simulink model "Task_2"  (R2021b)
settings: Solver=ode23tb  StartTime=0.0  StopTime=1000*3600  RelTol=1e-3
undefined symbols (not defined in the file): Ion, Lithium
libraries: eeStairGenerator x2, spsBatteryLib x1, spsControlledCurrentSourceLib x1, spspowerguiLib x1
settings Model: Creator=eee  LastModifiedBy=casum

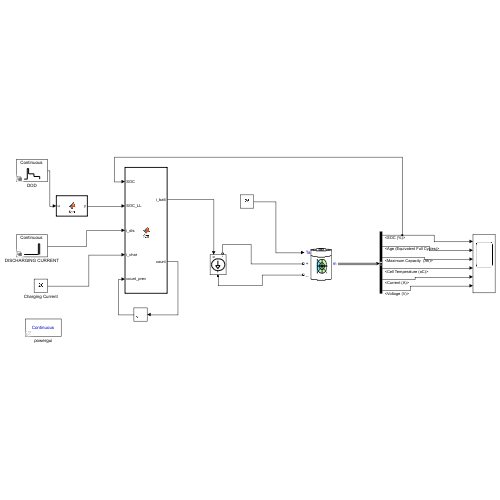
[thumbnail: Simulink's stored preview of the top-level diagram]
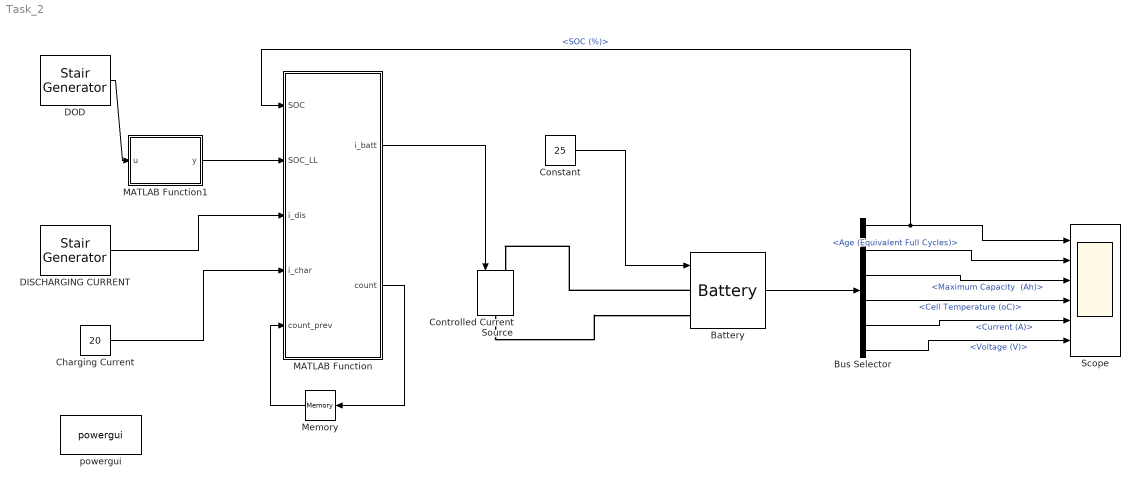
== system Task_2 ==
  Battery : spsBatteryLib/Battery  BatType=Lithium-Ion  ShowTempParam=on  ThermalPreset="12.8V  40Ah  (LiFeMgPO4)"  ShowAgeParam=on  NomV=12.6  NomQ=40  SOC=100  Batt_Tr=30  PresetModel=off  MaxQ=40  MinV=10.5  FullV=13.8  Dis_rate=20  R=0.015  Normal_OP=30.14  expZone="[13.1          0.5]"  current=[6.5 13 32.5]  Units=Time  Tci=25  NomT=20  T2=0  MaxQ2=36  FullV2=13  Normal_OP2=11.7  expZone2="[12.67            4]"  Rca=0.6411  ti=4880  Dp=0  Neq0=0  Tsim=30  Ta1=25  Qeol=40*0.9  Reol=0.013333*1.2  Char_age=[20, 30]  Dis_age=[20, 80]  N1=1500  N2=10500  N3=1000  N4=1400  Ta2=45  N5=950
  Bus Selector : BusSelector  OutputSignals="SOC (%),Age (Equivalent Full Cycles),Maximum Capacity  (Ah),Cell Temperature (oC),Current (A),Voltage (V)"
  Charging Current : Constant  Value=20
  Constant : Constant  Value=25
  Controlled Current Source : spsControlledCurrentSourceLib/Controlled Current Source  Initialize=on  Source_Type=AC  Amplitude=0  Phase=0  Frequency=0  Measurements=None
  DISCHARGING CURRENT : eeStairGenerator/Stair Generator  LabelModeActiveChoice=Continuous  TimeInput=[0 600*3600 650*3600]  AmplitudeInput=[20 80 20]  SampleTime=0  RepeatPattern=off  OutDataTypeStr=double
      settings: SourceProductBaseCode=PS
  DOD : eeStairGenerator/Stair Generator  LabelModeActiveChoice=Continuous  TimeInput=[0 175*3600 240*3600 540*3600 850*3600]  AmplitudeInput=[20 60 40 30 20]  SampleTime=0  RepeatPattern=off  OutDataTypeStr=double
      settings: SourceProductBaseCode=PS
  MATLAB Function : MATLAB Function  TreatAsAtomicUnit=on
  MATLAB Function1 : MATLAB Function  TreatAsAtomicUnit=on
  Memory : Memory  InitialCondition=1
  Scope : Scope  NumInputPorts=6
  powergui : spspowerguiLib/powergui  Priority=1  SimulationMode=Continuous  SampleTime=50e-6  frequency=60  Iterations=50  frequencyindice=0  Pbase=100e6  ErrMax=1e-4  UnitsV=kV  UnitsW=MW  buscounter=0  FunctionMessages=off  echomessages=off  EnableUseOfTLC=off  CurrentSourceSwitches=off  DisableSnubberDevices=off  DisableRonSwitches=off  DisableVfSwitches=off  DisplayEquations=off  AutomaticDiscreteSolvers=off  SolverType=Tustin/Backward Euler (TBE)  Interpol=off  ExternalGateDelay=off  methode=off  Ts=100  x0status=blocks  SPID=on  SwTol=0  HookPort=off  NonlinearTolerance=1e-4  nMaxIteration=100  ContinueOnMaxIteration=off  RestoreLinks=warning  ResistiveCurrentMeasurement=off  Frange=[0:2:500]  Ylog=off  Xlog=on  ShowGrid=off  save=off  variable=ZData  structure=0  ZoomFFT=off  StartTime=0.0  cycles=1  DisplayStyle=1  fundamental=60  FreqAxis=off  MaxFrequency=1000  frequencyindicesteady=1  RmsSteady=1  display=off
  wires:
  Constant/1 -> Battery/1
  Bus Selector/1 -> MATLAB Function/1(SOC), Scope/1  "<SOC (%)>"
  Bus Selector/2 -> Scope/2  "<Age (Equivalent Full Cycles)>"
  Bus Selector/3 -> Scope/3  "<Maximum Capacity  (Ah)>"
  Bus Selector/4 -> Scope/4  "<Cell Temperature (oC)>"
  Bus Selector/5 -> Scope/5  "<Current (A)>"
  Bus Selector/6 -> Scope/6  "<Voltage (V)>"
  Battery/1 -> Bus Selector/1
  MATLAB Function/2(count) -> Memory/1
  Memory/1 -> MATLAB Function/5(count_prev)
  Charging Current/1 -> MATLAB Function/4(i_char)
  DISCHARGING CURRENT/1 -> MATLAB Function/3(i_dis)
  MATLAB Function/1(i_batt) -> Controlled Current Source/1
  MATLAB Function1/1(y) -> MATLAB Function/2(SOC_LL)
  DOD/1 -> MATLAB Function1/1(u)
  connections:
  Battery/LConn1 -- Controlled Current Source/LConn1
  Controlled Current Source/RConn1 -- Battery/LConn2

== matlab function Task_2/MATLAB Function1 ==
  data: u input; y output
function y = fcn(u)
y = 100-u;
end

== matlab function Task_2/MATLAB Function ==
  data: SOC input; i_batt output; SOC_LL input; i_dis input; i_char input; count_prev input; count output
function [i_batt, count] = fcn(SOC, SOC_LL, i_dis, i_char, count_prev)
count=count_prev;
if(count_prev==1 && SOC<=SOC_LL)
    count=0;
end
if(count_prev==0 && SOC>=99)
   count=1;
end

if(count_prev==1)
   i_batt=i_dis;
else
    i_batt=-i_char;


end
